simulink model "Scratch3"  (Simulink 8.5)
settings: Solver=ode4  StartTime=0.0  StopTime=20  FixedStep=0.005  RelTol=1e-3
libraries: dspinverses x1, roblocks x1
(part 3 of 3)

== matlab function Gravity Matrix(G) ==
  data: G_Num output double; q1dd input double; q2dd input double; q3dd input double; q4dd input double; q1d input double; q2d input double; q3d input double; q4d input double; q1 input double; q2 input double; q3 input double; q4 input double; Gdot_Num output double; Gddot_Num output double
function [G_Num,Gdot_Num, Gddot_Num] = fcn(q1dd, q2dd, q3dd, q4dd, q1d, q2d, q3d, q4d, q1, q2, q3, q4)
%#codegen
% coder.extrinsic('evalin'); 
% coder.extrinsic('subs'); 
% coder.extrinsic('eval'); 
% 
% q_Sym = evalin('base','q');
% G_Sym = evalin('base','G');
% q_Num = [q1t;q2t;q3t;q4t];
% 
% Gdot_Sym = evalin('base','Gdot');
% States_Sym1 = evalin('base','states1');
% states1_Num = [q1t;q2t;q3t;q4t;q1dt;q2dt;q3dt;q4dt];
% 
% Gddot_Sym = evalin('base','Gddot');
% States_Sym2 = evalin('base','states2');
% states2_Num = [q1t;q2t;q3t;q4t;q1dt;q2dt;q3dt;q4dt;q1ddt;q2ddt;q3ddt;q4ddt];
% 
% G_Num = zeros(4,1);
% Gdot_Num = zeros(4,1);
% Gddot_Num = zeros(4,1);
% 
% G_Num = eval(subs(G_Sym,q_Sym,q_Num));
% Gdot_Num = eval(subs(Gdot_Sym,States_Sym1,states1_Num));
% Gddot_Num = eval(subs(Gddot_Sym,States_Sym2,states2_Num));

m1 = 10;
m2 = 7;
m3 = 7;
m4 = 5;
l1 = 1;
l2 = 0.7;
l3 = 0.7; 
l4 = 0.5;
d1 = l1/2;
d2 = l2/2;
d3 = l3/2; 
d4 = l4/2;
g0 = -9.81;

% G_Num = [g0*m3*(l2*cos(q1 + q2) + l1*cos(q1) + d3*cos(q1 + q2 + q3)) + g0*m2*(d2*cos(q1 + q2) + l1*cos(q1)) + g0*m4*(d4*cos(q1 + q2 + q3 + q4) + l2*cos(q1 + q2) + l1*cos(q1) + l3*cos(q1 + q2 + q3)) + d1*g0*m1*cos(q1)
%                                                              g0*m4*(d4*cos(q1 + q2 + q3 + q4) + l2*cos(q1 + q2) + l3*cos(q1 + q2 + q3)) + g0*m3*(l2*cos(q1 + q2) + d3*cos(q1 + q2 + q3)) + d2*g0*m2*cos(q1 + q2)
%                                                                                                                            g0*m4*(d4*cos(q1 + q2 + q3 + q4) + l3*cos(q1 + q2 + q3)) + d3*g0*m3*cos(q1 + q2 + q3)
%                                                                                                                                                                                  d4*g0*m4*cos(q1 + q2 + q3 + q4)];

G_Num = [- g0*m4*(d4*sin(q1 + q2 + q3 + q4) + l2*sin(q1 + q2) + l1*sin(q1) + l3*sin(q1 + q2 + q3)) - g0*m3*(l2*sin(q1 + q2) + l1*sin(q1) + d3*sin(q1 + q2 + q3)) - g0*m2*(d2*sin(q1 + q2) + l1*sin(q1)) - d1*g0*m1*sin(q1)
                                                             - g0*m4*(d4*sin(q1 + q2 + q3 + q4) + l2*sin(q1 + q2) + l3*sin(q1 + q2 + q3)) - g0*m3*(l2*sin(q1 + q2) + d3*sin(q1 + q2 + q3)) - d2*g0*m2*sin(q1 + q2)
                                                                                                                           - g0*m4*(d4*sin(q1 + q2 + q3 + q4) + l3*sin(q1 + q2 + q3)) - d3*g0*m3*sin(q1 + q2 + q3)
                                                                                                                                                                                  -d4*g0*m4*sin(q1 + q2 + q3 + q4)];


% Gdot_Num = [- q1d*(g0*m4*(d4*sin(q1 + q2 + q3 + q4) + l2*sin(q1 + q2) + l1*sin(q1) + l3*sin(q1 + q2 + q3)) + g0*m3*(l2*sin(q1 + q2) + l1*sin(q1) + d3*sin(q1 + q2 + q3)) + g0*m2*(d2*sin(q1 + q2) + l1*sin(q1)) + d1*g0*m1*sin(q1)) - q3d*(g0*m4*(d4*sin(q1 + q2 + q3 + q4) + l3*sin(q1 + q2 + q3)) + d3*g0*m3*sin(q1 + q2 + q3)) - q2d*(g0*m4*(d4*sin(q1 + q2 + q3 + q4) + l2*sin(q1 + q2) + l3*sin(q1 + q2 + q3)) + g0*m3*(l2*sin(q1 + q2) + d3*sin(q1 + q2 + q3)) + d2*g0*m2*sin(q1 + q2)) - d4*g0*m4*q4d*sin(q1 + q2 + q3 + q4)
%                                                              - q3d*(g0*m4*(d4*sin(q1 + q2 + q3 + q4) + l3*sin(q1 + q2 + q3)) + d3*g0*m3*sin(q1 + q2 + q3)) - q1d*(g0*m4*(d4*sin(q1 + q2 + q3 + q4) + l2*sin(q1 + q2) + l3*sin(q1 + q2 + q3)) + g0*m3*(l2*sin(q1 + q2) + d3*sin(q1 + q2 + q3)) + d2*g0*m2*sin(q1 + q2)) - q2d*(g0*m4*(d4*sin(q1 + q2 + q3 + q4) + l2*sin(q1 + q2) + l3*sin(q1 + q2 + q3)) + g0*m3*(l2*sin(q1 + q2) + d3*sin(q1 + q2 + q3)) + d2*g0*m2*sin(q1 + q2)) - d4*g0*m4*q4d*sin(q1 + q2 + q3 + q4)
%                                                                                                                                                                                          - q1d*(g0*m4*(d4*sin(q1 + q2 + q3 + q4) + l3*sin(q1 + q2 + q3)) + d3*g0*m3*sin(q1 + q2 + q3)) - q2d*(g0*m4*(d4*sin(q1 + q2 + q3 + q4) + l3*sin(q1 + q2 + q3)) + d3*g0*m3*sin(q1 + q2 + q3)) - q3d*(g0*m4*(d4*sin(q1 + q2 + q3 + q4) + l3*sin(q1 + q2 + q3)) + d3*g0*m3*sin(q1 + q2 + q3)) - d4*g0*m4*q4d*sin(q1 + q2 + q3 + q4)
%                                                                                                                                                                                                                                                                                                                                                                  - d4*g0*m4*q1d*sin(q1 + q2 + q3 + q4) - d4*g0*m4*q2d*sin(q1 + q2 + q3 + q4) - d4*g0*m4*q3d*sin(q1 + q2 + q3 + q4) - d4*g0*m4*q4d*sin(q1 + q2 + q3 + q4)];
%                                                                                                                                                                                                                                                                                                                                                              

Gdot_Num = [- q2d*(g0*m4*(d4*cos(q1 + q2 + q3 + q4) + l2*cos(q1 + q2) + l3*cos(q1 + q2 + q3)) + g0*m3*(l2*cos(q1 + q2) + d3*cos(q1 + q2 + q3)) + d2*g0*m2*cos(q1 + q2)) - q1d*(g0*m3*(l2*cos(q1 + q2) + l1*cos(q1) + d3*cos(q1 + q2 + q3)) + g0*m2*(d2*cos(q1 + q2) + l1*cos(q1)) + g0*m4*(d4*cos(q1 + q2 + q3 + q4) + l2*cos(q1 + q2) + l1*cos(q1) + l3*cos(q1 + q2 + q3)) + d1*g0*m1*cos(q1)) - q3d*(g0*m4*(d4*cos(q1 + q2 + q3 + q4) + l3*cos(q1 + q2 + q3)) + d3*g0*m3*cos(q1 + q2 + q3)) - d4*g0*m4*q4d*cos(q1 + q2 + q3 + q4)
                                                             - q1d*(g0*m4*(d4*cos(q1 + q2 + q3 + q4) + l2*cos(q1 + q2) + l3*cos(q1 + q2 + q3)) + g0*m3*(l2*cos(q1 + q2) + d3*cos(q1 + q2 + q3)) + d2*g0*m2*cos(q1 + q2)) - q2d*(g0*m4*(d4*cos(q1 + q2 + q3 + q4) + l2*cos(q1 + q2) + l3*cos(q1 + q2 + q3)) + g0*m3*(l2*cos(q1 + q2) + d3*cos(q1 + q2 + q3)) + d2*g0*m2*cos(q1 + q2)) - q3d*(g0*m4*(d4*cos(q1 + q2 + q3 + q4) + l3*cos(q1 + q2 + q3)) + d3*g0*m3*cos(q1 + q2 + q3)) - d4*g0*m4*q4d*cos(q1 + q2 + q3 + q4)
                                                                                                                                                                                         - q1d*(g0*m4*(d4*cos(q1 + q2 + q3 + q4) + l3*cos(q1 + q2 + q3)) + d3*g0*m3*cos(q1 + q2 + q3)) - q2d*(g0*m4*(d4*cos(q1 + q2 + q3 + q4) + l3*cos(q1 + q2 + q3)) + d3*g0*m3*cos(q1 + q2 + q3)) - q3d*(g0*m4*(d4*cos(q1 + q2 + q3 + q4) + l3*cos(q1 + q2 + q3)) + d3*g0*m3*cos(q1 + q2 + q3)) - d4*g0*m4*q4d*cos(q1 + q2 + q3 + q4)
                                                                                                                                                                                                                                                                                                                                                                 - d4*g0*m4*q1d*cos(q1 + q2 + q3 + q4) - d4*g0*m4*q2d*cos(q1 + q2 + q3 + q4) - d4*g0*m4*q3d*cos(q1 + q2 + q3 + q4) - d4*g0*m4*q4d*cos(q1 + q2 + q3 + q4)];
                                                                                                                                                                                                                                                                                                                                                             
                                                                                                                                                                                                                                                                                                                                                             
% Gddot_Num = [- d2*g0*m2*q1d^2*cos(q1 + q2) - d2*g0*m2*q2d^2*cos(q1 + q2) - g0*l2*m3*q1d^2*cos(q1 + q2) - g0*l2*m3*q2d^2*cos(q1 + q2) - g0*l2*m4*q1d^2*cos(q1 + q2) - g0*l2*m4*q2d^2*cos(q1 + q2) - d3*g0*m3*q1dd*sin(q1 + q2 + q3) - d3*g0*m3*q2dd*sin(q1 + q2 + q3) - d3*g0*m3*q3dd*sin(q1 + q2 + q3) - g0*l3*m4*q1dd*sin(q1 + q2 + q3) - g0*l3*m4*q2dd*sin(q1 + q2 + q3) - g0*l3*m4*q3dd*sin(q1 + q2 + q3) - d1*g0*m1*q1d^2*cos(q1) - g0*l1*m2*q1d^2*cos(q1) - g0*l1*m3*q1d^2*cos(q1) - g0*l1*m4*q1d^2*cos(q1) - d3*g0*m3*q1d^2*cos(q1 + q2 + q3) - d3*g0*m3*q2d^2*cos(q1 + q2 + q3) - d3*g0*m3*q3d^2*cos(q1 + q2 + q3) - g0*l3*m4*q1d^2*cos(q1 + q2 + q3) - g0*l3*m4*q2d^2*cos(q1 + q2 + q3) - g0*l3*m4*q3d^2*cos(q1 + q2 + q3) - d4*g0*m4*q1dd*sin(q1 + q2 + q3 + q4) - d4*g0*m4*q2dd*sin(q1 + q2 + q3 + q4) - d4*g0*m4*q3dd*sin(q1 + q2 + q3 + q4) - d4*g0*m4*q4dd*sin(q1 + q2 + q3 + q4) - d2*g0*m2*q1dd*sin(q1 + q2) - d2*g0*m2*q2dd*sin(q1 + q2) - g0*l2*m3*q1dd*sin(q1 + q2) - g0*l2*m3*q2dd*sin(q1 + q2) - g0*l2*m4*q1dd*sin(q1 + q2) - g0*l2*m4*q2dd*sin(q1 + q2) - d1*g0*m1*q1dd*sin(q1) - d4*g0*m4*q1d^2*cos(q1 + q2 + q3 + q4) - d4*g0*m4*q2d^2*cos(q1 + q2 + q3 + q4) - d4*g0*m4*q3d^2*cos(q1 + q2 + q3 + q4) - d4*g0*m4*q4d^2*cos(q1 + q2 + q3 + q4) - g0*l1*m2*q1dd*sin(q1) - g0*l1*m3*q1dd*sin(q1) - g0*l1*m4*q1dd*sin(q1) - 2*d4*g0*m4*q1d*q2d*cos(q1 + q2 + q3 + q4) - 2*d4*g0*m4*q1d*q3d*cos(q1 + q2 + q3 + q4) - 2*d4*g0*m4*q1d*q4d*cos(q1 + q2 + q3 + q4) - 2*d4*g0*m4*q2d*q3d*cos(q1 + q2 + q3 + q4) - 2*d4*g0*m4*q2d*q4d*cos(q1 + q2 + q3 + q4) - 2*d4*g0*m4*q3d*q4d*cos(q1 + q2 + q3 + q4) - 2*d2*g0*m2*q1d*q2d*cos(q1 + q2) - 2*g0*l2*m3*q1d*q2d*cos(q1 + q2) - 2*g0*l2*m4*q1d*q2d*cos(q1 + q2) - 2*d3*g0*m3*q1d*q2d*cos(q1 + q2 + q3) - 2*d3*g0*m3*q1d*q3d*cos(q1 + q2 + q3) - 2*d3*g0*m3*q2d*q3d*cos(q1 + q2 + q3) - 2*g0*l3*m4*q1d*q2d*cos(q1 + q2 + q3) - 2*g0*l3*m4*q1d*q3d*cos(q1 + q2 + q3) - 2*g0*l3*m4*q2d*q3d*cos(q1 + q2 + q3)
%                                                                                                                                                                                                      - d2*g0*m2*q1d^2*cos(q1 + q2) - d2*g0*m2*q2d^2*cos(q1 + q2) - g0*l2*m3*q1d^2*cos(q1 + q2) - g0*l2*m3*q2d^2*cos(q1 + q2) - g0*l2*m4*q1d^2*cos(q1 + q2) - g0*l2*m4*q2d^2*cos(q1 + q2) - d3*g0*m3*q1dd*sin(q1 + q2 + q3) - d3*g0*m3*q2dd*sin(q1 + q2 + q3) - d3*g0*m3*q3dd*sin(q1 + q2 + q3) - g0*l3*m4*q1dd*sin(q1 + q2 + q3) - g0*l3*m4*q2dd*sin(q1 + q2 + q3) - g0*l3*m4*q3dd*sin(q1 + q2 + q3) - d3*g0*m3*q1d^2*cos(q1 + q2 + q3) - d3*g0*m3*q2d^2*cos(q1 + q2 + q3) - d3*g0*m3*q3d^2*cos(q1 + q2 + q3) - g0*l3*m4*q1d^2*cos(q1 + q2 + q3) - g0*l3*m4*q2d^2*cos(q1 + q2 + q3) - g0*l3*m4*q3d^2*cos(q1 + q2 + q3) - d4*g0*m4*q1dd*sin(q1 + q2 + q3 + q4) - d4*g0*m4*q2dd*sin(q1 + q2 + q3 + q4) - d4*g0*m4*q3dd*sin(q1 + q2 + q3 + q4) - d4*g0*m4*q4dd*sin(q1 + q2 + q3 + q4) - d2*g0*m2*q1dd*sin(q1 + q2) - d2*g0*m2*q2dd*sin(q1 + q2) - g0*l2*m3*q1dd*sin(q1 + q2) - g0*l2*m3*q2dd*sin(q1 + q2) - g0*l2*m4*q1dd*sin(q1 + q2) - g0*l2*m4*q2dd*sin(q1 + q2) - d4*g0*m4*q1d^2*cos(q1 + q2 + q3 + q4) - d4*g0*m4*q2d^2*cos(q1 + q2 + q3 + q4) - d4*g0*m4*q3d^2*cos(q1 + q2 + q3 + q4) - d4*g0*m4*q4d^2*cos(q1 + q2 + q3 + q4) - 2*d4*g0*m4*q1d*q2d*cos(q1 + q2 + q3 + q4) - 2*d4*g0*m4*q1d*q3d*cos(q1 + q2 + q3 + q4) - 2*d4*g0*m4*q1d*q4d*cos(q1 + q2 + q3 + q4) - 2*d4*g0*m4*q2d*q3d*cos(q1 + q2 + q3 + q4) - 2*d4*g0*m4*q2d*q4d*cos(q1 + q2 + q3 + q4) - 2*d4*g0*m4*q3d*q4d*cos(q1 + q2 + q3 + q4) - 2*d2*g0*m2*q1d*q2d*cos(q1 + q2) - 2*g0*l2*m3*q1d*q2d*cos(q1 + q2) - 2*g0*l2*m4*q1d*q2d*cos(q1 + q2) - 2*d3*g0*m3*q1d*q2d*cos(q1 + q2 + q3) - 2*d3*g0*m3*q1d*q3d*cos(q1 + q2 + q3) - 2*d3*g0*m3*q2d*q3d*cos(q1 + q2 + q3) - 2*g0*l3*m4*q1d*q2d*cos(q1 + q2 + q3) - 2*g0*l3*m4*q1d*q3d*cos(q1 + q2 + q3) - 2*g0*l3*m4*q2d*q3d*cos(q1 + q2 + q3)
%                                                                                                                                                                                                                                                                                                                                                                                                                                                                                                                                                                                                                                                                              - d3*g0*m3*q1dd*sin(q1 + q2 + q3) - d3*g0*m3*q2dd*sin(q1 + q2 + q3) - d3*g0*m3*q3dd*sin(q1 + q2 + q3) - g0*l3*m4*q1dd*sin(q1 + q2 + q3) - g0*l3*m4*q2dd*sin(q1 + q2 + q3) - g0*l3*m4*q3dd*sin(q1 + q2 + q3) - d3*g0*m3*q1d^2*cos(q1 + q2 + q3) - d3*g0*m3*q2d^2*cos(q1 + q2 + q3) - d3*g0*m3*q3d^2*cos(q1 + q2 + q3) - g0*l3*m4*q1d^2*cos(q1 + q2 + q3) - g0*l3*m4*q2d^2*cos(q1 + q2 + q3) - g0*l3*m4*q3d^2*cos(q1 + q2 + q3) - d4*g0*m4*q1dd*sin(q1 + q2 + q3 + q4) - d4*g0*m4*q2dd*sin(q1 + q2 + q3 + q4) - d4*g0*m4*q3dd*sin(q1 + q2 + q3 + q4) - d4*g0*m4*q4dd*sin(q1 + q2 + q3 + q4) - d4*g0*m4*q1d^2*cos(q1 + q2 + q3 + q4) - d4*g0*m4*q2d^2*cos(q1 + q2 + q3 + q4) - d4*g0*m4*q3d^2*cos(q1 + q2 + q3 + q4) - d4*g0*m4*q4d^2*cos(q1 + q2 + q3 + q4) - 2*d4*g0*m4*q1d*q2d*cos(q1 + q2 + q3 + q4) - 2*d4*g0*m4*q1d*q3d*cos(q1 + q2 + q3 + q4) - 2*d4*g0*m4*q1d*q4d*cos(q1 + q2 + q3 + q4) - 2*d4*g0*m4*q2d*q3d*cos(q1 + q2 + q3 + q4) - 2*d4*g0*m4*q2d*q4d*cos(q1 + q2 + q3 + q4) - 2*d4*g0*m4*q3d*q4d*cos(q1 + q2 + q3 + q4) - 2*d3*g0*m3*q1d*q2d*cos(q1 + q2 + q3) - 2*d3*g0*m3*q1d*q3d*cos(q1 + q2 + q3) - 2*d3*g0*m3*q2d*q3d*cos(q1 + q2 + q3) - 2*g0*l3*m4*q1d*q2d*cos(q1 + q2 + q3) - 2*g0*l3*m4*q1d*q3d*cos(q1 + q2 + q3) - 2*g0*l3*m4*q2d*q3d*cos(q1 + q2 + q3)
%                                                                                                                                                                                                                                                                                                                                                                                                                                                                                                                                                                                                                                                                                                                                                                                                                                                                                                                                                                                                                                                                                                                                                                                                                                                                                                                                                                                                                                                                                                                                                                                                                                    - d4*g0*m4*sin(q1 + q2 + q3 + q4)*(q1dd + q2dd + q3dd + q4dd) - d4*g0*m4*q1d*cos(q1 + q2 + q3 + q4)*(q1d + q2d + q3d + q4d) - d4*g0*m4*q2d*cos(q1 + q2 + q3 + q4)*(q1d + q2d + q3d + q4d) - d4*g0*m4*q3d*cos(q1 + q2 + q3 + q4)*(q1d + q2d + q3d + q4d) - d4*g0*m4*q4d*cos(q1 + q2 + q3 + q4)*(q1d + q2d + q3d + q4d)];


Gddot_Num = [ d2*g0*m2*q1d^2*sin(q1 + q2) + d2*g0*m2*q2d^2*sin(q1 + q2) - d3*g0*m3*q1dd*cos(q1 + q2 + q3) - d3*g0*m3*q2dd*cos(q1 + q2 + q3) - d3*g0*m3*q3dd*cos(q1 + q2 + q3) + g0*l2*m3*q1d^2*sin(q1 + q2) + g0*l2*m3*q2d^2*sin(q1 + q2) + g0*l2*m4*q1d^2*sin(q1 + q2) + g0*l2*m4*q2d^2*sin(q1 + q2) - g0*l3*m4*q1dd*cos(q1 + q2 + q3) - g0*l3*m4*q2dd*cos(q1 + q2 + q3) - g0*l3*m4*q3dd*cos(q1 + q2 + q3) + d1*g0*m1*q1d^2*sin(q1) + g0*l1*m2*q1d^2*sin(q1) + g0*l1*m3*q1d^2*sin(q1) + g0*l1*m4*q1d^2*sin(q1) + d3*g0*m3*q1d^2*sin(q1 + q2 + q3) + d3*g0*m3*q2d^2*sin(q1 + q2 + q3) + d3*g0*m3*q3d^2*sin(q1 + q2 + q3) - d4*g0*m4*q1dd*cos(q1 + q2 + q3 + q4) - d4*g0*m4*q2dd*cos(q1 + q2 + q3 + q4) - d4*g0*m4*q3dd*cos(q1 + q2 + q3 + q4) - d4*g0*m4*q4dd*cos(q1 + q2 + q3 + q4) + g0*l3*m4*q1d^2*sin(q1 + q2 + q3) + g0*l3*m4*q2d^2*sin(q1 + q2 + q3) + g0*l3*m4*q3d^2*sin(q1 + q2 + q3) - d2*g0*m2*q1dd*cos(q1 + q2) - d2*g0*m2*q2dd*cos(q1 + q2) - g0*l2*m3*q1dd*cos(q1 + q2) - g0*l2*m3*q2dd*cos(q1 + q2) - g0*l2*m4*q1dd*cos(q1 + q2) - g0*l2*m4*q2dd*cos(q1 + q2) - d1*g0*m1*q1dd*cos(q1) - g0*l1*m2*q1dd*cos(q1) - g0*l1*m3*q1dd*cos(q1) - g0*l1*m4*q1dd*cos(q1) + d4*g0*m4*q1d^2*sin(q1 + q2 + q3 + q4) + d4*g0*m4*q2d^2*sin(q1 + q2 + q3 + q4) + d4*g0*m4*q3d^2*sin(q1 + q2 + q3 + q4) + d4*g0*m4*q4d^2*sin(q1 + q2 + q3 + q4) + 2*d4*g0*m4*q1d*q2d*sin(q1 + q2 + q3 + q4) + 2*d4*g0*m4*q1d*q3d*sin(q1 + q2 + q3 + q4) + 2*d4*g0*m4*q1d*q4d*sin(q1 + q2 + q3 + q4) + 2*d4*g0*m4*q2d*q3d*sin(q1 + q2 + q3 + q4) + 2*d4*g0*m4*q2d*q4d*sin(q1 + q2 + q3 + q4) + 2*d4*g0*m4*q3d*q4d*sin(q1 + q2 + q3 + q4) + 2*d2*g0*m2*q1d*q2d*sin(q1 + q2) + 2*g0*l2*m3*q1d*q2d*sin(q1 + q2) + 2*g0*l2*m4*q1d*q2d*sin(q1 + q2) + 2*d3*g0*m3*q1d*q2d*sin(q1 + q2 + q3) + 2*d3*g0*m3*q1d*q3d*sin(q1 + q2 + q3) + 2*d3*g0*m3*q2d*q3d*sin(q1 + q2 + q3) + 2*g0*l3*m4*q1d*q2d*sin(q1 + q2 + q3) + 2*g0*l3*m4*q1d*q3d*sin(q1 + q2 + q3) + 2*g0*l3*m4*q2d*q3d*sin(q1 + q2 + q3)
                                                                                                                                                                                                     d2*g0*m2*q1d^2*sin(q1 + q2) + d2*g0*m2*q2d^2*sin(q1 + q2) - d3*g0*m3*q1dd*cos(q1 + q2 + q3) - d3*g0*m3*q2dd*cos(q1 + q2 + q3) - d3*g0*m3*q3dd*cos(q1 + q2 + q3) + g0*l2*m3*q1d^2*sin(q1 + q2) + g0*l2*m3*q2d^2*sin(q1 + q2) + g0*l2*m4*q1d^2*sin(q1 + q2) + g0*l2*m4*q2d^2*sin(q1 + q2) - g0*l3*m4*q1dd*cos(q1 + q2 + q3) - g0*l3*m4*q2dd*cos(q1 + q2 + q3) - g0*l3*m4*q3dd*cos(q1 + q2 + q3) + d3*g0*m3*q1d^2*sin(q1 + q2 + q3) + d3*g0*m3*q2d^2*sin(q1 + q2 + q3) + d3*g0*m3*q3d^2*sin(q1 + q2 + q3) - d4*g0*m4*q1dd*cos(q1 + q2 + q3 + q4) - d4*g0*m4*q2dd*cos(q1 + q2 + q3 + q4) - d4*g0*m4*q3dd*cos(q1 + q2 + q3 + q4) - d4*g0*m4*q4dd*cos(q1 + q2 + q3 + q4) + g0*l3*m4*q1d^2*sin(q1 + q2 + q3) + g0*l3*m4*q2d^2*sin(q1 + q2 + q3) + g0*l3*m4*q3d^2*sin(q1 + q2 + q3) - d2*g0*m2*q1dd*cos(q1 + q2) - d2*g0*m2*q2dd*cos(q1 + q2) - g0*l2*m3*q1dd*cos(q1 + q2) - g0*l2*m3*q2dd*cos(q1 + q2) - g0*l2*m4*q1dd*cos(q1 + q2) - g0*l2*m4*q2dd*cos(q1 + q2) + d4*g0*m4*q1d^2*sin(q1 + q2 + q3 + q4) + d4*g0*m4*q2d^2*sin(q1 + q2 + q3 + q4) + d4*g0*m4*q3d^2*sin(q1 + q2 + q3 + q4) + d4*g0*m4*q4d^2*sin(q1 + q2 + q3 + q4) + 2*d4*g0*m4*q1d*q2d*sin(q1 + q2 + q3 + q4) + 2*d4*g0*m4*q1d*q3d*sin(q1 + q2 + q3 + q4) + 2*d4*g0*m4*q1d*q4d*sin(q1 + q2 + q3 + q4) + 2*d4*g0*m4*q2d*q3d*sin(q1 + q2 + q3 + q4) + 2*d4*g0*m4*q2d*q4d*sin(q1 + q2 + q3 + q4) + 2*d4*g0*m4*q3d*q4d*sin(q1 + q2 + q3 + q4) + 2*d2*g0*m2*q1d*q2d*sin(q1 + q2) + 2*g0*l2*m3*q1d*q2d*sin(q1 + q2) + 2*g0*l2*m4*q1d*q2d*sin(q1 + q2) + 2*d3*g0*m3*q1d*q2d*sin(q1 + q2 + q3) + 2*d3*g0*m3*q1d*q3d*sin(q1 + q2 + q3) + 2*d3*g0*m3*q2d*q3d*sin(q1 + q2 + q3) + 2*g0*l3*m4*q1d*q2d*sin(q1 + q2 + q3) + 2*g0*l3*m4*q1d*q3d*sin(q1 + q2 + q3) + 2*g0*l3*m4*q2d*q3d*sin(q1 + q2 + q3)
                                                                                                                                                                                                                                                                                                                                                                                                                                                                                                                                                                                                                                                                             d3*g0*m3*q1d^2*sin(q1 + q2 + q3) - d3*g0*m3*q2dd*cos(q1 + q2 + q3) - d3*g0*m3*q3dd*cos(q1 + q2 + q3) - g0*l3*m4*q1dd*cos(q1 + q2 + q3) - g0*l3*m4*q2dd*cos(q1 + q2 + q3) - g0*l3*m4*q3dd*cos(q1 + q2 + q3) - d3*g0*m3*q1dd*cos(q1 + q2 + q3) + d3*g0*m3*q2d^2*sin(q1 + q2 + q3) + d3*g0*m3*q3d^2*sin(q1 + q2 + q3) - d4*g0*m4*q1dd*cos(q1 + q2 + q3 + q4) - d4*g0*m4*q2dd*cos(q1 + q2 + q3 + q4) - d4*g0*m4*q3dd*cos(q1 + q2 + q3 + q4) - d4*g0*m4*q4dd*cos(q1 + q2 + q3 + q4) + g0*l3*m4*q1d^2*sin(q1 + q2 + q3) + g0*l3*m4*q2d^2*sin(q1 + q2 + q3) + g0*l3*m4*q3d^2*sin(q1 + q2 + q3) + d4*g0*m4*q1d^2*sin(q1 + q2 + q3 + q4) + d4*g0*m4*q2d^2*sin(q1 + q2 + q3 + q4) + d4*g0*m4*q3d^2*sin(q1 + q2 + q3 + q4) + d4*g0*m4*q4d^2*sin(q1 + q2 + q3 + q4) + 2*d4*g0*m4*q1d*q2d*sin(q1 + q2 + q3 + q4) + 2*d4*g0*m4*q1d*q3d*sin(q1 + q2 + q3 + q4) + 2*d4*g0*m4*q1d*q4d*sin(q1 + q2 + q3 + q4) + 2*d4*g0*m4*q2d*q3d*sin(q1 + q2 + q3 + q4) + 2*d4*g0*m4*q2d*q4d*sin(q1 + q2 + q3 + q4) + 2*d4*g0*m4*q3d*q4d*sin(q1 + q2 + q3 + q4) + 2*d3*g0*m3*q1d*q2d*sin(q1 + q2 + q3) + 2*d3*g0*m3*q1d*q3d*sin(q1 + q2 + q3) + 2*d3*g0*m3*q2d*q3d*sin(q1 + q2 + q3) + 2*g0*l3*m4*q1d*q2d*sin(q1 + q2 + q3) + 2*g0*l3*m4*q1d*q3d*sin(q1 + q2 + q3) + 2*g0*l3*m4*q2d*q3d*sin(q1 + q2 + q3)
                                                                                                                                                                                                                                                                                                                                                                                                                                                                                                                                                                                                                                                                                                                                                                                                                                                                                                                                                                                                                                                                                                                                                                                                                                                                                                                                                                                                                                                                                                                                                                                                                                   d4*g0*m4*q1d*sin(q1 + q2 + q3 + q4)*(q1d + q2d + q3d + q4d) - d4*g0*m4*cos(q1 + q2 + q3 + q4)*(q1dd + q2dd + q3dd + q4dd) + d4*g0*m4*q2d*sin(q1 + q2 + q3 + q4)*(q1d + q2d + q3d + q4d) + d4*g0*m4*q3d*sin(q1 + q2 + q3 + q4)*(q1d + q2d + q3d + q4d) + d4*g0*m4*q4d*sin(q1 + q2 + q3 + q4)*(q1d + q2d + q3d + q4d)];
